simulink model "simulacao"  (R2018a)
settings: Solver=VariableStepAuto  StartTime=0.0  StopTime=10.0  RelTol=1e-3
settings Model: Creator=aluno  LastModifiedBy=aluno

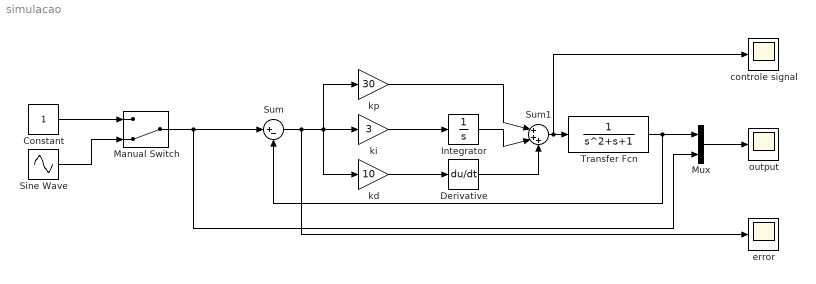
== system simulacao ==
  Constant : Constant
  Derivative : Derivative
  Integrator : Integrator
  Manual Switch : ManualSwitch  CurrentSetting=0
  Mux : Mux  Inputs=2
  Sine Wave : Sin  SampleTime=0
  Sum : Sum  Inputs=|+-
  Sum1 : Sum  Inputs=|+++
  Transfer Fcn : TransferFcn  Denominator=[1 1 1]
  controle signal : Scope
  error : Scope
  kd : Gain  Gain=10
  ki : Gain  Gain=3
  kp : Gain  Gain=30
  output : Scope
  wires:
  Mux/1 -> output/1
  Sum/1 -> error/1, kp/1, ki/1, kd/1
  Transfer Fcn/1 -> Sum/2, Mux/1
  kd/1 -> Derivative/1
  ki/1 -> Integrator/1
  kp/1 -> Sum1/1
  Integrator/1 -> Sum1/2
  Derivative/1 -> Sum1/3
  Sum1/1 -> controle signal/1, Transfer Fcn/1
  Manual Switch/1 -> Mux/2, Sum/1
  Constant/1 -> Manual Switch/1
  Sine Wave/1 -> Manual Switch/2
